simulink model "BEM_theory_harness"  (R2020b)
settings: Solver=ode4  StartTime=0.0  StopTime=par.sym.Ttot  MaxStep=par.sym.max_dt  RelTol=1e-3  SampleTimeConstraint=STIndependent
settings Model: Creator=carar  LastModifiedBy=carar
settings SolverCC: AlgebraicLoopSolver=LineSearch
settings DataIOCC: SaveOutput=off  SaveTime=off  ReturnWorkspaceOutputs=off  TimeSaveName=TIME
settings OptimizationCC: LifeSpan=inf
settings DebuggingCC: UnconnectedInputMsg=none  UnconnectedOutputMsg=none  ArithmeticOperatorsInVariantConditions=warning
settings SFSimCC: CustomCodeUndefinedFunction=UseInterfaceOnly
settings CodeAppCC: GenerateComments=off
settings SimscapeCC: SimscapeNormalizeSystem=off

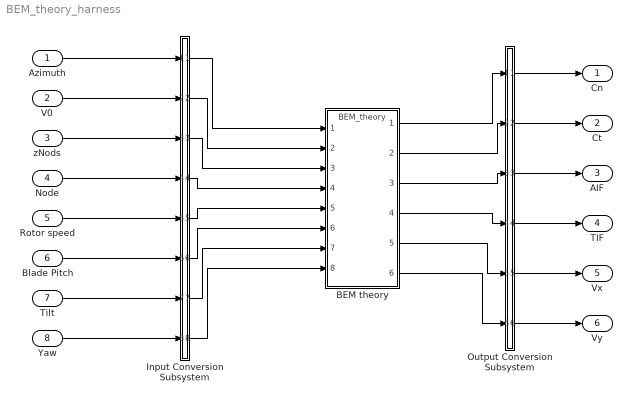
== system BEM_theory_harness ==
  Azimuth : Inport  OutDataTypeStr=double  PortDimensions=[1]
  V0 : Inport  Port=2  OutDataTypeStr=double  PortDimensions=[3]
  zNods : Inport  Port=3  OutDataTypeStr=double  PortDimensions=[1]
  Node : Inport  Port=4  OutDataTypeStr=double  PortDimensions=[1]
  Rotor speed : Inport  Port=5  OutDataTypeStr=double  PortDimensions=[1]
  Blade Pitch : Inport  Port=6  OutDataTypeStr=double  PortDimensions=[1]
  Tilt : Inport  Port=7  OutDataTypeStr=double  PortDimensions=[1]
  Yaw : Inport  Port=8  OutDataTypeStr=double  PortDimensions=[1]
  BEM theory : ModelReference  ModelNameDialog=BEM_theory.slxp  ModelReferenceVersion=5.17  CopyOfModelProtected=on
  Input Conversion Subsystem : Subsystem  Tag=__SLT_ICS__  Description=|
      | Signal spec.
      | and routing
      settings: AttributesFormatString=%<Description>
  Output Conversion Subsystem : Subsystem  Tag=__SLT_OCS__  Description=|
      | Signal spec.
      | and routing
      settings: AttributesFormatString=%<Description>
  Cn : Outport
  Ct : Outport  Port=2
  AIF : Outport  Port=3
  TIF : Outport  Port=4
  Vx : Outport  Port=5
  Vy : Outport  Port=6
  wires:
  Azimuth/1 -> Input Conversion Subsystem/1(Inport_1)
  V0/1 -> Input Conversion Subsystem/2(Inport_2)
  zNods/1 -> Input Conversion Subsystem/3(Inport_3)
  Node/1 -> Input Conversion Subsystem/4(Inport_4)
  Rotor speed/1 -> Input Conversion Subsystem/5(Inport_5)
  Blade Pitch/1 -> Input Conversion Subsystem/6(Inport_6)
  Tilt/1 -> Input Conversion Subsystem/7(Inport_7)
  Yaw/1 -> Input Conversion Subsystem/8(Inport_8)
  Output Conversion Subsystem/1(Outport_1) -> Cn/1
  Output Conversion Subsystem/2(Outport_2) -> Ct/1
  Output Conversion Subsystem/3(Outport_3) -> AIF/1
  Output Conversion Subsystem/4(Outport_4) -> TIF/1
  Output Conversion Subsystem/5(Outport_5) -> Vx/1
  Output Conversion Subsystem/6(Outport_6) -> Vy/1
  Input Conversion Subsystem/1(Outport_1) -> BEM theory/1
  Input Conversion Subsystem/2(Outport_2) -> BEM theory/2
  Input Conversion Subsystem/3(Outport_3) -> BEM theory/3
  Input Conversion Subsystem/4(Outport_4) -> BEM theory/4
  Input Conversion Subsystem/5(Outport_5) -> BEM theory/5
  Input Conversion Subsystem/6(Outport_6) -> BEM theory/6
  Input Conversion Subsystem/7(Outport_7) -> BEM theory/7
  Input Conversion Subsystem/8(Outport_8) -> BEM theory/8
  BEM theory/1 -> Output Conversion Subsystem/1(Inport_1)
  BEM theory/2 -> Output Conversion Subsystem/2(Inport_2)
  BEM theory/3 -> Output Conversion Subsystem/3(Inport_3)
  BEM theory/4 -> Output Conversion Subsystem/4(Inport_4)
  BEM theory/5 -> Output Conversion Subsystem/5(Inport_5)
  BEM theory/6 -> Output Conversion Subsystem/6(Inport_6)

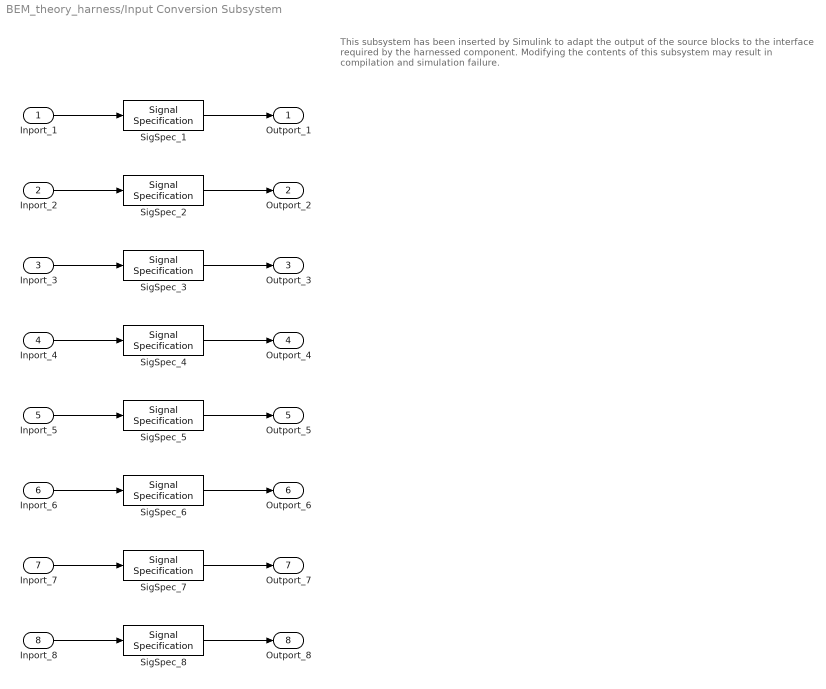
== system BEM_theory_harness/Input Conversion Subsystem ==
  note: This subsystem has been inserted by Simulink to adapt the output of the source blocks to the interface required by the harnessed component.
      |  Modifying the contents of this subsystem may result in compilation and simulation failure.
  Inport_1 : Inport
  Inport_2 : Inport  Port=2
  Inport_3 : Inport  Port=3
  Inport_4 : Inport  Port=4
  Inport_5 : Inport  Port=5
  Inport_6 : Inport  Port=6
  Inport_7 : Inport  Port=7
  Inport_8 : Inport  Port=8
  SigSpec_{1,3..8} (7 alike) : SignalSpecification  OutDataTypeStr=double  Dimensions=[1]
  SigSpec_2 : SignalSpecification  OutDataTypeStr=double  Dimensions=[3]
  Outport_1 : Outport
  Outport_2 : Outport  Port=2
  Outport_3 : Outport  Port=3
  Outport_4 : Outport  Port=4
  Outport_5 : Outport  Port=5
  Outport_6 : Outport  Port=6
  Outport_7 : Outport  Port=7
  Outport_8 : Outport  Port=8
  wires:
  SigSpec_1/1 -> Outport_1/1
  Inport_1/1 -> SigSpec_1/1
  SigSpec_2/1 -> Outport_2/1
  Inport_2/1 -> SigSpec_2/1
  SigSpec_3/1 -> Outport_3/1
  Inport_3/1 -> SigSpec_3/1
  SigSpec_4/1 -> Outport_4/1
  Inport_4/1 -> SigSpec_4/1
  SigSpec_5/1 -> Outport_5/1
  Inport_5/1 -> SigSpec_5/1
  SigSpec_6/1 -> Outport_6/1
  Inport_6/1 -> SigSpec_6/1
  SigSpec_7/1 -> Outport_7/1
  Inport_7/1 -> SigSpec_7/1
  SigSpec_8/1 -> Outport_8/1
  Inport_8/1 -> SigSpec_8/1

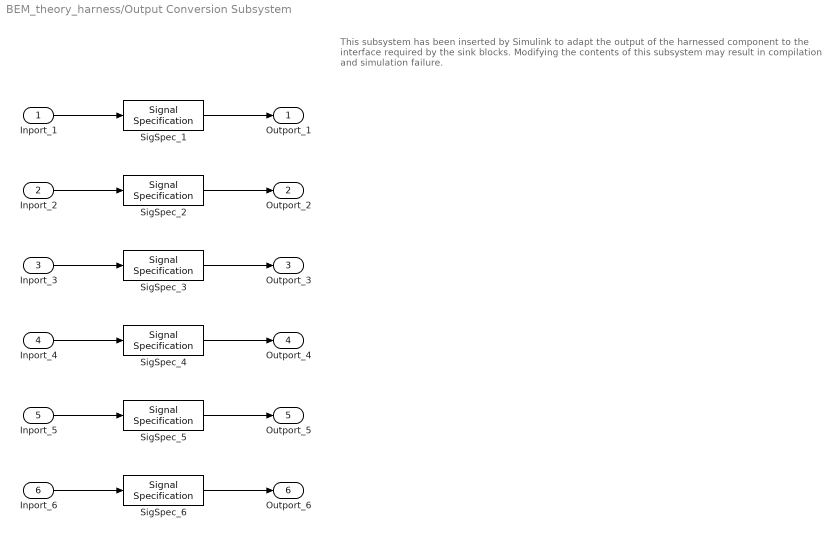
== system BEM_theory_harness/Output Conversion Subsystem ==
  note: This subsystem has been inserted by Simulink to adapt the output of the harnessed component to the interface required by the sink blocks.
      |  Modifying the contents of this subsystem may result in compilation and simulation failure.
  Inport_1 : Inport
  Inport_2 : Inport  Port=2
  Inport_3 : Inport  Port=3
  Inport_4 : Inport  Port=4
  Inport_5 : Inport  Port=5
  Inport_6 : Inport  Port=6
  SigSpec_{1..6} (6 alike) : SignalSpecification  OutDataTypeStr=double  Dimensions=[1]
  Outport_1 : Outport
  Outport_2 : Outport  Port=2
  Outport_3 : Outport  Port=3
  Outport_4 : Outport  Port=4
  Outport_5 : Outport  Port=5
  Outport_6 : Outport  Port=6
  wires:
  Inport_1/1 -> SigSpec_1/1
  SigSpec_1/1 -> Outport_1/1
  Inport_2/1 -> SigSpec_2/1
  SigSpec_2/1 -> Outport_2/1
  Inport_3/1 -> SigSpec_3/1
  SigSpec_3/1 -> Outport_3/1
  Inport_4/1 -> SigSpec_4/1
  SigSpec_4/1 -> Outport_4/1
  Inport_5/1 -> SigSpec_5/1
  SigSpec_5/1 -> Outport_5/1
  Inport_6/1 -> SigSpec_6/1
  SigSpec_6/1 -> Outport_6/1
